simulink model "gm_parallel_phase_voltages_per_switching_state_6"  (R2022a)
settings: Solver=FixedStepDiscrete  StartTime=0.0  StopTime=10.0  RelTol=1e-3
undefined symbols (not defined in the file or in its folder): f_c, u_dc
libraries: hdlmdlgenlib x82
(part 4 of 5)

== system gm_parallel_phase_voltages_per_switching_state_6/Phase_voltages_per_switching_state/Subsystem/MATLAB Function7 ==
  theta_el_with_offset : Inport  OutDataTypeStr=single  PortDimensions=1  SampleTime=1e-08
  u_dc_link_voltage : Inport  Port=2  OutDataTypeStr=single  PortDimensions=1  SampleTime=1e-08
  Index : Inport  Port=3  OutDataTypeStr=int32  PortDimensions=1  SampleTime=1e-08
  Assignment : Assignment  NumberOfDimensions=2  SampleTime=1e-08  IndexOptions=Index vector (dialog),Index vector (dialog)  Indices=double(2),double(1)  OutputSizes=double(0),double(0)
  Assignment1 : Assignment  NumberOfDimensions=2  SampleTime=1e-08  IndexOptions=Index vector (dialog),Index vector (dialog)  Indices=double(1),double(1)  OutputSizes=double(0),double(0)
  Assignment2 : Assignment  NumberOfDimensions=2  SampleTime=1e-08  IndexOptions=Index vector (dialog),Index vector (dialog)  Indices=double(4),double(1)  OutputSizes=double(0),double(0)
  Assignment3 : Assignment  NumberOfDimensions=2  SampleTime=1e-08  IndexOptions=Index vector (dialog),Index vector (dialog)  Indices=double(3),double(1)  OutputSizes=double(0),double(0)
  Selector : Selector  NumberOfDimensions=2  SampleTime=1e-08  IndexOptions=Index vector (dialog),Index vector (dialog)  Indices=double(1),double(1)  OutputSizes=double(0),double(0)
  Selector1 : Selector  NumberOfDimensions=2  SampleTime=1e-08  IndexOptions=Index vector (dialog),Index vector (dialog)  Indices=double(2),double(1)  OutputSizes=double(0),double(0)
  Selector2 : Selector  NumberOfDimensions=2  SampleTime=1e-08  IndexOptions=Index vector (dialog),Index vector (dialog)  Indices=double(3),double(1)  OutputSizes=double(0),double(0)
  Selector3 : Selector  NumberOfDimensions=2  SampleTime=1e-08  IndexOptions=Index vector (dialog),Index vector (dialog)  Indices=double(4),double(1)  OutputSizes=double(0),double(0)
  Selector4 : Selector  NumberOfDimensions=2  SampleTime=1e-08  IndexOptions=Index vector (dialog),Index vector (port)  Indices=double(2),double(-1)  OutputSizes=double(0),double(0)
  Selector5 : Selector  NumberOfDimensions=2  SampleTime=1e-08  IndexOptions=Index vector (dialog),Index vector (port)  Indices=double(1),double(-1)  OutputSizes=double(0),double(0)
  Selector6 : Selector  NumberOfDimensions=2  SampleTime=1e-08  IndexOptions=Index vector (dialog),Index vector (port)  Indices=double(4),double(-1)  OutputSizes=double(0),double(0)
  Selector7 : Selector  NumberOfDimensions=2  SampleTime=1e-08  IndexOptions=Index vector (dialog),Index vector (port)  Indices=double(2),double(-1)  OutputSizes=double(0),double(0)
  Selector8 : Selector  NumberOfDimensions=2  SampleTime=1e-08  IndexOptions=Index vector (dialog),Index vector (port)  Indices=double(1),double(-1)  OutputSizes=double(0),double(0)
  Selector9 : Selector  NumberOfDimensions=2  SampleTime=1e-08  IndexOptions=Index vector (dialog),Index vector (port)  Indices=double(3),double(-1)  OutputSizes=double(0),double(0)
  adder : Sum  AccumDataTypeStr=int32  OutDataTypeStr=int32  RndMeth=Nearest  SaturateOnIntegerOverflow=on  SampleTime=1e-08
  adder1 : Subsystem
      mask Display: disp('NFP\nadd');
  adder2 : Subsystem
      mask Display: disp('NFP\nadd');
  const{,1..2,5..7} (6 alike) : Constant  Value=single([0 -0.3333333432674408 0 -0.3333333432674408 0.3333333432674408 -0.3333333432674408 0.3333333432674408 -0.3333333432674408 -0.1666666716337204 -0.044658198952674866 -0.1666666716337204 -0.6220084428787231 0.1666666716337204 -0.044658198952674866 0.1666666716337204 -0.6220084428787231]).'  VectorParams1D=off  OutDataTypeStr=single  SampleTime=1e-08
  const3 : Constant  Value="repmat(single(0),[4  1])"  VectorParams1D=off  OutDataTypeStr=single  SampleTime=1e-08
  const4 : Constant  VectorParams1D=off  OutDataTypeStr=int32  SampleTime=1e-08
  cos_to_sincos : Subsystem
      mask Display: disp('NFP\ntrig2');
  cos_to_sincos_out1_buff : hdlmdlgenlib/Buffer
      settings: SourceProductBaseCode=SL
  cos_to_sincos_out2_buff : hdlmdlgenlib/Buffer
      settings: SourceProductBaseCode=SL
  delayMatch{,1,3..4} (4 alike) : Delay  DelayLength=double(27)  InitialCondition=0  SampleTime=1e-08
  delayMatch{6..11} (6 alike) : Delay  DelayLength=double(2)  InitialCondition=0  SampleTime=1e-08
  delayMatch{12..17} (6 alike) : Delay  DelayLength=double(16)  InitialCondition=0  SampleTime=1e-08
  delayMatch2 : Delay  DelayLength=double(39)  InitialCondition=0  SampleTime=1e-08
  delayMatch5 : Delay  DelayLength=double(39)  InitialCondition=0  SampleTime=1e-08
  multiplier : Subsystem
      mask Display: disp('NFP\nmul');
  multiplier1 : Subsystem
      mask Display: disp('NFP\nmul');
  multiplier2 : Subsystem
      mask Display: disp('NFP\nmul');
  multiplier3 : Subsystem
      mask Display: disp('NFP\nmul');
  multiplier4 : Subsystem
      mask Display: disp('NFP\nmul');
  multiplier_outbuff : hdlmdlgenlib/Buffer
      settings: SourceProductBaseCode=SL
  t{,1..5} (6 alike) : Reshape  OutputDimensionality=Customize  OutputDimensions=[4,4]
  t6 : Mux
  uminus : Subsystem
      mask Display: disp('NFP\numinus');
  d_voltage_per_switching_state : Outport  SampleTime=1e-08  VectorParamsAs1DForOutWhenUnconnected=off
  q_voltage_per_switching_state : Outport  Port=2  SampleTime=1e-08
  x_voltage_per_switching_state : Outport  Port=3  SampleTime=1e-08
  y_voltage_per_switching_state : Outport  Port=4  SampleTime=1e-08
  wires:
  Selector/1 -> d_voltage_per_switching_state/1
  Selector1/1 -> q_voltage_per_switching_state/1
  Selector2/1 -> x_voltage_per_switching_state/1
  Selector3/1 -> y_voltage_per_switching_state/1
  multiplier_outbuff/1 -> Selector3/1, Selector2/1, Selector1/1, Selector/1
  Assignment/1 -> multiplier/2(In2)
  Assignment1/1 -> Assignment/1
  delayMatch14/1 -> Assignment1/1
  delayMatch16/1 -> multiplier1/2(In2)
  cos_to_sincos_out2_buff/1 -> multiplier4/1(In1), multiplier1/1(In1)
  delayMatch15/1 -> multiplier2/2(In2)
  Selector6/1 -> Assignment2/2
  Assignment3/1 -> Assignment2/1
  adder/1 -> Selector9/2, Selector8/2, Selector7/2, Selector6/2, Selector5/2, Selector4/2
  t/1 -> Selector4/1
  t1/1 -> Selector5/1
  cos_to_sincos_out1_buff/1 -> multiplier3/1(In1), uminus/1(In1)
  delayMatch13/1 -> multiplier3/2(In2)
  delayMatch12/1 -> multiplier4/2(In2)
  t2/1 -> Selector6/1
  Selector9/1 -> Assignment3/2
  const3/1 -> Assignment3/1
  const4/1 -> adder/2
  t3/1 -> Selector7/1
  t4/1 -> Selector8/1
  t5/1 -> Selector9/1
  const/1 -> t/1
  const1/1 -> t1/1
  const2/1 -> t2/1
  const5/1 -> t3/1
  const6/1 -> t4/1
  const7/1 -> t5/1
  delayMatch17/1 -> multiplier/1(In1)
  multiplier/1(Out1) -> multiplier_outbuff/1
  adder1/1(Out1) -> Assignment/2
  multiplier1/1(Out1) -> adder1/2(In2)
  multiplier2/1(Out1) -> adder1/1(In1)
  adder2/1(Out1) -> Assignment1/2
  uminus/1(Out1) -> multiplier2/1(In1)
  multiplier3/1(Out1) -> adder2/2(In2)
  multiplier4/1(Out1) -> adder2/1(In1)
  cos_to_sincos/1(Out1) -> cos_to_sincos_out1_buff/1
  cos_to_sincos/2(Out2) -> cos_to_sincos_out2_buff/1
  Selector8/1 -> delayMatch/1
  Selector7/1 -> delayMatch1/1
  Assignment2/1 -> delayMatch2/1
  Selector5/1 -> delayMatch3/1
  Selector4/1 -> delayMatch4/1
  t6/1 -> delayMatch5/1
  delayMatch/1 -> delayMatch6/1
  delayMatch1/1 -> delayMatch7/1
  delayMatch2/1 -> delayMatch8/1
  delayMatch3/1 -> delayMatch9/1
  delayMatch4/1 -> delayMatch10/1
  delayMatch5/1 -> delayMatch11/1
  delayMatch6/1 -> delayMatch12/1
  delayMatch7/1 -> delayMatch13/1
  delayMatch8/1 -> delayMatch14/1
  delayMatch9/1 -> delayMatch15/1
  delayMatch10/1 -> delayMatch16/1
  delayMatch11/1 -> delayMatch17/1
  theta_el_with_offset/1 -> cos_to_sincos/1(In1)
  u_dc_link_voltage/1 -> t6/4, t6/3, t6/2, t6/1
  Index/1 -> adder/1

== system gm_parallel_phase_voltages_per_switching_state_6/Phase_voltages_per_switching_state/Subsystem/MATLAB Function8 ==
  theta_el_with_offset : Inport  OutDataTypeStr=single  PortDimensions=1  SampleTime=1e-08
  u_dc_link_voltage : Inport  Port=2  OutDataTypeStr=single  PortDimensions=1  SampleTime=1e-08
  Index : Inport  Port=3  OutDataTypeStr=int32  PortDimensions=1  SampleTime=1e-08
  Assignment : Assignment  NumberOfDimensions=2  SampleTime=1e-08  IndexOptions=Index vector (dialog),Index vector (dialog)  Indices=double(2),double(1)  OutputSizes=double(0),double(0)
  Assignment1 : Assignment  NumberOfDimensions=2  SampleTime=1e-08  IndexOptions=Index vector (dialog),Index vector (dialog)  Indices=double(1),double(1)  OutputSizes=double(0),double(0)
  Assignment2 : Assignment  NumberOfDimensions=2  SampleTime=1e-08  IndexOptions=Index vector (dialog),Index vector (dialog)  Indices=double(4),double(1)  OutputSizes=double(0),double(0)
  Assignment3 : Assignment  NumberOfDimensions=2  SampleTime=1e-08  IndexOptions=Index vector (dialog),Index vector (dialog)  Indices=double(3),double(1)  OutputSizes=double(0),double(0)
  Selector : Selector  NumberOfDimensions=2  SampleTime=1e-08  IndexOptions=Index vector (dialog),Index vector (dialog)  Indices=double(1),double(1)  OutputSizes=double(0),double(0)
  Selector1 : Selector  NumberOfDimensions=2  SampleTime=1e-08  IndexOptions=Index vector (dialog),Index vector (dialog)  Indices=double(2),double(1)  OutputSizes=double(0),double(0)
  Selector2 : Selector  NumberOfDimensions=2  SampleTime=1e-08  IndexOptions=Index vector (dialog),Index vector (dialog)  Indices=double(3),double(1)  OutputSizes=double(0),double(0)
  Selector3 : Selector  NumberOfDimensions=2  SampleTime=1e-08  IndexOptions=Index vector (dialog),Index vector (dialog)  Indices=double(4),double(1)  OutputSizes=double(0),double(0)
  Selector4 : Selector  NumberOfDimensions=2  SampleTime=1e-08  IndexOptions=Index vector (dialog),Index vector (port)  Indices=double(2),double(-1)  OutputSizes=double(0),double(0)
  Selector5 : Selector  NumberOfDimensions=2  SampleTime=1e-08  IndexOptions=Index vector (dialog),Index vector (port)  Indices=double(1),double(-1)  OutputSizes=double(0),double(0)
  Selector6 : Selector  NumberOfDimensions=2  SampleTime=1e-08  IndexOptions=Index vector (dialog),Index vector (port)  Indices=double(4),double(-1)  OutputSizes=double(0),double(0)
  Selector7 : Selector  NumberOfDimensions=2  SampleTime=1e-08  IndexOptions=Index vector (dialog),Index vector (port)  Indices=double(2),double(-1)  OutputSizes=double(0),double(0)
  Selector8 : Selector  NumberOfDimensions=2  SampleTime=1e-08  IndexOptions=Index vector (dialog),Index vector (port)  Indices=double(1),double(-1)  OutputSizes=double(0),double(0)
  Selector9 : Selector  NumberOfDimensions=2  SampleTime=1e-08  IndexOptions=Index vector (dialog),Index vector (port)  Indices=double(3),double(-1)  OutputSizes=double(0),double(0)
  adder : Sum  AccumDataTypeStr=int32  OutDataTypeStr=int32  RndMeth=Nearest  SaturateOnIntegerOverflow=on  SampleTime=1e-08
  adder1 : Subsystem
      mask Display: disp('NFP\nadd');
  adder2 : Subsystem
      mask Display: disp('NFP\nadd');
  const{,1..2,5..7} (6 alike) : Constant  Value=single([-0.1666666716337204 0.044658198952674866 -0.1666666716337204 0.6220084428787231 0.1666666716337204 0.044658198952674866 0.1666666716337204 0.6220084428787231 -0.3333333432674408 0.3333333432674408 -0.3333333432674408 0.3333333432674408 0 0.3333333432674408 0 0.3333333432674408]).'  VectorParams1D=off  OutDataTypeStr=single  SampleTime=1e-08
  const3 : Constant  Value="repmat(single(0),[4  1])"  VectorParams1D=off  OutDataTypeStr=single  SampleTime=1e-08
  const4 : Constant  VectorParams1D=off  OutDataTypeStr=int32  SampleTime=1e-08
  cos_to_sincos : Subsystem
      mask Display: disp('NFP\ntrig2');
  cos_to_sincos_out1_buff : hdlmdlgenlib/Buffer
      settings: SourceProductBaseCode=SL
  cos_to_sincos_out2_buff : hdlmdlgenlib/Buffer
      settings: SourceProductBaseCode=SL
  delayMatch{,1,3..4} (4 alike) : Delay  DelayLength=double(27)  InitialCondition=0  SampleTime=1e-08
  delayMatch{6..11} (6 alike) : Delay  DelayLength=double(2)  InitialCondition=0  SampleTime=1e-08
  delayMatch{12..17} (6 alike) : Delay  DelayLength=double(16)  InitialCondition=0  SampleTime=1e-08
  delayMatch2 : Delay  DelayLength=double(39)  InitialCondition=0  SampleTime=1e-08
  delayMatch5 : Delay  DelayLength=double(39)  InitialCondition=0  SampleTime=1e-08
  multiplier : Subsystem
      mask Display: disp('NFP\nmul');
  multiplier1 : Subsystem
      mask Display: disp('NFP\nmul');
  multiplier2 : Subsystem
      mask Display: disp('NFP\nmul');
  multiplier3 : Subsystem
      mask Display: disp('NFP\nmul');
  multiplier4 : Subsystem
      mask Display: disp('NFP\nmul');
  multiplier_outbuff : hdlmdlgenlib/Buffer
      settings: SourceProductBaseCode=SL
  t{,1..5} (6 alike) : Reshape  OutputDimensionality=Customize  OutputDimensions=[4,4]
  t6 : Mux
  uminus : Subsystem
      mask Display: disp('NFP\numinus');
  d_voltage_per_switching_state : Outport  SampleTime=1e-08  VectorParamsAs1DForOutWhenUnconnected=off
  q_voltage_per_switching_state : Outport  Port=2  SampleTime=1e-08
  x_voltage_per_switching_state : Outport  Port=3  SampleTime=1e-08
  y_voltage_per_switching_state : Outport  Port=4  SampleTime=1e-08
  wires:
  Selector/1 -> d_voltage_per_switching_state/1
  Selector1/1 -> q_voltage_per_switching_state/1
  Selector2/1 -> x_voltage_per_switching_state/1
  Selector3/1 -> y_voltage_per_switching_state/1
  multiplier_outbuff/1 -> Selector3/1, Selector2/1, Selector1/1, Selector/1
  Assignment/1 -> multiplier/2(In2)
  Assignment1/1 -> Assignment/1
  delayMatch14/1 -> Assignment1/1
  delayMatch16/1 -> multiplier1/2(In2)
  cos_to_sincos_out2_buff/1 -> multiplier4/1(In1), multiplier1/1(In1)
  delayMatch15/1 -> multiplier2/2(In2)
  Selector6/1 -> Assignment2/2
  Assignment3/1 -> Assignment2/1
  adder/1 -> Selector9/2, Selector8/2, Selector7/2, Selector6/2, Selector5/2, Selector4/2
  t/1 -> Selector4/1
  t1/1 -> Selector5/1
  cos_to_sincos_out1_buff/1 -> multiplier3/1(In1), uminus/1(In1)
  delayMatch13/1 -> multiplier3/2(In2)
  delayMatch12/1 -> multiplier4/2(In2)
  t2/1 -> Selector6/1
  Selector9/1 -> Assignment3/2
  const3/1 -> Assignment3/1
  const4/1 -> adder/2
  t3/1 -> Selector7/1
  t4/1 -> Selector8/1
  t5/1 -> Selector9/1
  const/1 -> t/1
  const1/1 -> t1/1
  const2/1 -> t2/1
  const5/1 -> t3/1
  const6/1 -> t4/1
  const7/1 -> t5/1
  delayMatch17/1 -> multiplier/1(In1)
  multiplier/1(Out1) -> multiplier_outbuff/1
  adder1/1(Out1) -> Assignment/2
  multiplier1/1(Out1) -> adder1/2(In2)
  multiplier2/1(Out1) -> adder1/1(In1)
  adder2/1(Out1) -> Assignment1/2
  uminus/1(Out1) -> multiplier2/1(In1)
  multiplier3/1(Out1) -> adder2/2(In2)
  multiplier4/1(Out1) -> adder2/1(In1)
  cos_to_sincos/1(Out1) -> cos_to_sincos_out1_buff/1
  cos_to_sincos/2(Out2) -> cos_to_sincos_out2_buff/1
  Selector8/1 -> delayMatch/1
  Selector7/1 -> delayMatch1/1
  Assignment2/1 -> delayMatch2/1
  Selector5/1 -> delayMatch3/1
  Selector4/1 -> delayMatch4/1
  t6/1 -> delayMatch5/1
  delayMatch/1 -> delayMatch6/1
  delayMatch1/1 -> delayMatch7/1
  delayMatch2/1 -> delayMatch8/1
  delayMatch3/1 -> delayMatch9/1
  delayMatch4/1 -> delayMatch10/1
  delayMatch5/1 -> delayMatch11/1
  delayMatch6/1 -> delayMatch12/1
  delayMatch7/1 -> delayMatch13/1
  delayMatch8/1 -> delayMatch14/1
  delayMatch9/1 -> delayMatch15/1
  delayMatch10/1 -> delayMatch16/1
  delayMatch11/1 -> delayMatch17/1
  theta_el_with_offset/1 -> cos_to_sincos/1(In1)
  u_dc_link_voltage/1 -> t6/4, t6/3, t6/2, t6/1
  Index/1 -> adder/1

== system gm_parallel_phase_voltages_per_switching_state_6/Phase_voltages_per_switching_state/Subsystem/MATLAB Function9 ==
  theta_el_with_offset : Inport  OutDataTypeStr=single  PortDimensions=1  SampleTime=1e-08
  u_dc_link_voltage : Inport  Port=2  OutDataTypeStr=single  PortDimensions=1  SampleTime=1e-08
  Index : Inport  Port=3  OutDataTypeStr=int32  PortDimensions=1  SampleTime=1e-08
  Assignment : Assignment  NumberOfDimensions=2  SampleTime=1e-08  IndexOptions=Index vector (dialog),Index vector (dialog)  Indices=double(2),double(1)  OutputSizes=double(0),double(0)
  Assignment1 : Assignment  NumberOfDimensions=2  SampleTime=1e-08  IndexOptions=Index vector (dialog),Index vector (dialog)  Indices=double(1),double(1)  OutputSizes=double(0),double(0)
  Assignment2 : Assignment  NumberOfDimensions=2  SampleTime=1e-08  IndexOptions=Index vector (dialog),Index vector (dialog)  Indices=double(4),double(1)  OutputSizes=double(0),double(0)
  Assignment3 : Assignment  NumberOfDimensions=2  SampleTime=1e-08  IndexOptions=Index vector (dialog),Index vector (dialog)  Indices=double(3),double(1)  OutputSizes=double(0),double(0)
  Selector : Selector  NumberOfDimensions=2  SampleTime=1e-08  IndexOptions=Index vector (dialog),Index vector (dialog)  Indices=double(1),double(1)  OutputSizes=double(0),double(0)
  Selector1 : Selector  NumberOfDimensions=2  SampleTime=1e-08  IndexOptions=Index vector (dialog),Index vector (dialog)  Indices=double(2),double(1)  OutputSizes=double(0),double(0)
  Selector2 : Selector  NumberOfDimensions=2  SampleTime=1e-08  IndexOptions=Index vector (dialog),Index vector (dialog)  Indices=double(3),double(1)  OutputSizes=double(0),double(0)
  Selector3 : Selector  NumberOfDimensions=2  SampleTime=1e-08  IndexOptions=Index vector (dialog),Index vector (dialog)  Indices=double(4),double(1)  OutputSizes=double(0),double(0)
  Selector4 : Selector  NumberOfDimensions=2  SampleTime=1e-08  IndexOptions=Index vector (dialog),Index vector (port)  Indices=double(2),double(-1)  OutputSizes=double(0),double(0)
  Selector5 : Selector  NumberOfDimensions=2  SampleTime=1e-08  IndexOptions=Index vector (dialog),Index vector (port)  Indices=double(1),double(-1)  OutputSizes=double(0),double(0)
  Selector6 : Selector  NumberOfDimensions=2  SampleTime=1e-08  IndexOptions=Index vector (dialog),Index vector (port)  Indices=double(4),double(-1)  OutputSizes=double(0),double(0)
  Selector7 : Selector  NumberOfDimensions=2  SampleTime=1e-08  IndexOptions=Index vector (dialog),Index vector (port)  Indices=double(2),double(-1)  OutputSizes=double(0),double(0)
  Selector8 : Selector  NumberOfDimensions=2  SampleTime=1e-08  IndexOptions=Index vector (dialog),Index vector (port)  Indices=double(1),double(-1)  OutputSizes=double(0),double(0)
  Selector9 : Selector  NumberOfDimensions=2  SampleTime=1e-08  IndexOptions=Index vector (dialog),Index vector (port)  Indices=double(3),double(-1)  OutputSizes=double(0),double(0)
  adder : Sum  AccumDataTypeStr=int32  OutDataTypeStr=int32  RndMeth=Nearest  SaturateOnIntegerOverflow=on  SampleTime=1e-08
  adder1 : Subsystem
      mask Display: disp('NFP\nadd');
  adder2 : Subsystem
      mask Display: disp('NFP\nadd');
  const{,1..2,5..7} (6 alike) : Constant  Value=single([0 0.3333333432674408 0 0.3333333432674408 0.3333333432674408 0.3333333432674408 0.3333333432674408 0.3333333432674408 -0.1666666716337204 0.6220084428787231 -0.1666666716337204 0.044658198952674866 0.1666666716337204 0.6220084428787231 0.1666666716337204 0.044658198952674866]).'  VectorParams1D=off  OutDataTypeStr=single  SampleTime=1e-08
  const3 : Constant  Value="repmat(single(0),[4  1])"  VectorParams1D=off  OutDataTypeStr=single  SampleTime=1e-08
  const4 : Constant  VectorParams1D=off  OutDataTypeStr=int32  SampleTime=1e-08
  cos_to_sincos : Subsystem
      mask Display: disp('NFP\ntrig2');
  cos_to_sincos_out1_buff : hdlmdlgenlib/Buffer
      settings: SourceProductBaseCode=SL
  cos_to_sincos_out2_buff : hdlmdlgenlib/Buffer
      settings: SourceProductBaseCode=SL
  delayMatch{,1,3..4} (4 alike) : Delay  DelayLength=double(27)  InitialCondition=0  SampleTime=1e-08
  delayMatch{6..11} (6 alike) : Delay  DelayLength=double(2)  InitialCondition=0  SampleTime=1e-08
  delayMatch{12..17} (6 alike) : Delay  DelayLength=double(16)  InitialCondition=0  SampleTime=1e-08
  delayMatch2 : Delay  DelayLength=double(39)  InitialCondition=0  SampleTime=1e-08
  delayMatch5 : Delay  DelayLength=double(39)  InitialCondition=0  SampleTime=1e-08
  multiplier : Subsystem
      mask Display: disp('NFP\nmul');
  multiplier1 : Subsystem
      mask Display: disp('NFP\nmul');
  multiplier2 : Subsystem
      mask Display: disp('NFP\nmul');
  multiplier3 : Subsystem
      mask Display: disp('NFP\nmul');
  multiplier4 : Subsystem
      mask Display: disp('NFP\nmul');
  multiplier_outbuff : hdlmdlgenlib/Buffer
      settings: SourceProductBaseCode=SL
  t{,1..5} (6 alike) : Reshape  OutputDimensionality=Customize  OutputDimensions=[4,4]
  t6 : Mux
  uminus : Subsystem
      mask Display: disp('NFP\numinus');
  d_voltage_per_switching_state : Outport  SampleTime=1e-08  VectorParamsAs1DForOutWhenUnconnected=off
  q_voltage_per_switching_state : Outport  Port=2  SampleTime=1e-08
  x_voltage_per_switching_state : Outport  Port=3  SampleTime=1e-08
  y_voltage_per_switching_state : Outport  Port=4  SampleTime=1e-08
  wires:
  Selector/1 -> d_voltage_per_switching_state/1
  Selector1/1 -> q_voltage_per_switching_state/1
  Selector2/1 -> x_voltage_per_switching_state/1
  Selector3/1 -> y_voltage_per_switching_state/1
  multiplier_outbuff/1 -> Selector3/1, Selector2/1, Selector1/1, Selector/1
  Assignment/1 -> multiplier/2(In2)
  Assignment1/1 -> Assignment/1
  delayMatch14/1 -> Assignment1/1
  delayMatch16/1 -> multiplier1/2(In2)
  cos_to_sincos_out2_buff/1 -> multiplier4/1(In1), multiplier1/1(In1)
  delayMatch15/1 -> multiplier2/2(In2)
  Selector6/1 -> Assignment2/2
  Assignment3/1 -> Assignment2/1
  adder/1 -> Selector9/2, Selector8/2, Selector7/2, Selector6/2, Selector5/2, Selector4/2
  t/1 -> Selector4/1
  t1/1 -> Selector5/1
  cos_to_sincos_out1_buff/1 -> multiplier3/1(In1), uminus/1(In1)
  delayMatch13/1 -> multiplier3/2(In2)
  delayMatch12/1 -> multiplier4/2(In2)
  t2/1 -> Selector6/1
  Selector9/1 -> Assignment3/2
  const3/1 -> Assignment3/1
  const4/1 -> adder/2
  t3/1 -> Selector7/1
  t4/1 -> Selector8/1
  t5/1 -> Selector9/1
  const/1 -> t/1
  const1/1 -> t1/1
  const2/1 -> t2/1
  const5/1 -> t3/1
  const6/1 -> t4/1
  const7/1 -> t5/1
  delayMatch17/1 -> multiplier/1(In1)
  multiplier/1(Out1) -> multiplier_outbuff/1
  adder1/1(Out1) -> Assignment/2
  multiplier1/1(Out1) -> adder1/2(In2)
  multiplier2/1(Out1) -> adder1/1(In1)
  adder2/1(Out1) -> Assignment1/2
  uminus/1(Out1) -> multiplier2/1(In1)
  multiplier3/1(Out1) -> adder2/2(In2)
  multiplier4/1(Out1) -> adder2/1(In1)
  cos_to_sincos/1(Out1) -> cos_to_sincos_out1_buff/1
  cos_to_sincos/2(Out2) -> cos_to_sincos_out2_buff/1
  Selector8/1 -> delayMatch/1
  Selector7/1 -> delayMatch1/1
  Assignment2/1 -> delayMatch2/1
  Selector5/1 -> delayMatch3/1
  Selector4/1 -> delayMatch4/1
  t6/1 -> delayMatch5/1
  delayMatch/1 -> delayMatch6/1
  delayMatch1/1 -> delayMatch7/1
  delayMatch2/1 -> delayMatch8/1
  delayMatch3/1 -> delayMatch9/1
  delayMatch4/1 -> delayMatch10/1
  delayMatch5/1 -> delayMatch11/1
  delayMatch6/1 -> delayMatch12/1
  delayMatch7/1 -> delayMatch13/1
  delayMatch8/1 -> delayMatch14/1
  delayMatch9/1 -> delayMatch15/1
  delayMatch10/1 -> delayMatch16/1
  delayMatch11/1 -> delayMatch17/1
  theta_el_with_offset/1 -> cos_to_sincos/1(In1)
  u_dc_link_voltage/1 -> t6/4, t6/3, t6/2, t6/1
  Index/1 -> adder/1

== system gm_parallel_phase_voltages_per_switching_state_6/Phase_voltages_per_switching_state/Subsystem/MATLAB Function/adder1 ==
  In1 : Inport
  In2 : Inport  Port=2
  adder1 : Sum  OutDataTypeStr=single  SampleTime=1e-08
  adder1_pd1 : Delay  DelayLength=6
  Out1 : Outport
  wires:
  In1/1 -> adder1/1
  In2/1 -> adder1/2
  adder1/1 -> adder1_pd1/1
  adder1_pd1/1 -> Out1/1

== system gm_parallel_phase_voltages_per_switching_state_6/Phase_voltages_per_switching_state/Subsystem/MATLAB Function/adder2 ==
  In1 : Inport
  In2 : Inport  Port=2
  adder2 : Sum  OutDataTypeStr=single  SampleTime=1e-08
  adder2_pd1 : Delay  DelayLength=6
  Out1 : Outport
  wires:
  In1/1 -> adder2/1
  In2/1 -> adder2/2
  adder2/1 -> adder2_pd1/1
  adder2_pd1/1 -> Out1/1

== system gm_parallel_phase_voltages_per_switching_state_6/Phase_voltages_per_switching_state/Subsystem/MATLAB Function/cos_to_sincos ==
  In1 : Inport
  cos_to_sincos : Trigonometry  Operator=sincos  SampleTime=1e-08
  cos_to_sincos_pd1 : Delay  DelayLength=27
  cos_to_sincos_pd2 : Delay  DelayLength=27
  Out1 : Outport
  Out2 : Outport  Port=2
  wires:
  In1/1 -> cos_to_sincos/1
  cos_to_sincos/1 -> cos_to_sincos_pd1/1
  cos_to_sincos_pd1/1 -> Out1/1
  cos_to_sincos/2 -> cos_to_sincos_pd2/1
  cos_to_sincos_pd2/1 -> Out2/1

== system gm_parallel_phase_voltages_per_switching_state_6/Phase_voltages_per_switching_state/Subsystem/MATLAB Function/multiplier ==
  In1 : Inport
  In2 : Inport  Port=2
  multiplier : Product  Inputs=**  OutDataTypeStr=single  SampleTime=1e-08
  multiplier_pd1 : Delay  DelayLength=6
  Out1 : Outport
  wires:
  In1/1 -> multiplier/1
  In2/1 -> multiplier/2
  multiplier/1 -> multiplier_pd1/1
  multiplier_pd1/1 -> Out1/1

== system gm_parallel_phase_voltages_per_switching_state_6/Phase_voltages_per_switching_state/Subsystem/MATLAB Function/multiplier1 ==
  In1 : Inport
  In2 : Inport  Port=2
  multiplier1 : Product  Inputs=**  OutDataTypeStr=single  SampleTime=1e-08
  multiplier1_pd1 : Delay  DelayLength=6
  Out1 : Outport
  wires:
  In1/1 -> multiplier1/1
  In2/1 -> multiplier1/2
  multiplier1/1 -> multiplier1_pd1/1
  multiplier1_pd1/1 -> Out1/1

== system gm_parallel_phase_voltages_per_switching_state_6/Phase_voltages_per_switching_state/Subsystem/MATLAB Function/multiplier2 ==
  In1 : Inport
  In2 : Inport  Port=2
  multiplier2 : Product  Inputs=**  OutDataTypeStr=single  SampleTime=1e-08
  multiplier2_pd1 : Delay  DelayLength=6
  Out1 : Outport
  wires:
  In1/1 -> multiplier2/1
  In2/1 -> multiplier2/2
  multiplier2/1 -> multiplier2_pd1/1
  multiplier2_pd1/1 -> Out1/1

== system gm_parallel_phase_voltages_per_switching_state_6/Phase_voltages_per_switching_state/Subsystem/MATLAB Function/multiplier3 ==
  In1 : Inport
  In2 : Inport  Port=2
  multiplier3 : Product  Inputs=**  OutDataTypeStr=single  SampleTime=1e-08
  multiplier3_pd1 : Delay  DelayLength=6
  Out1 : Outport
  wires:
  In1/1 -> multiplier3/1
  In2/1 -> multiplier3/2
  multiplier3/1 -> multiplier3_pd1/1
  multiplier3_pd1/1 -> Out1/1

== system gm_parallel_phase_voltages_per_switching_state_6/Phase_voltages_per_switching_state/Subsystem/MATLAB Function/multiplier4 ==
  In1 : Inport
  In2 : Inport  Port=2
  multiplier4 : Product  Inputs=**  OutDataTypeStr=single  SampleTime=1e-08
  multiplier4_pd1 : Delay  DelayLength=6
  Out1 : Outport
  wires:
  In1/1 -> multiplier4/1
  In2/1 -> multiplier4/2
  multiplier4/1 -> multiplier4_pd1/1
  multiplier4_pd1/1 -> Out1/1

== system gm_parallel_phase_voltages_per_switching_state_6/Phase_voltages_per_switching_state/Subsystem/MATLAB Function/uminus ==
  In1 : Inport
  uminus : UnaryMinus  SampleTime=1e-08
  Out1 : Outport
  wires:
  In1/1 -> uminus/1
  uminus/1 -> Out1/1

== system gm_parallel_phase_voltages_per_switching_state_6/Phase_voltages_per_switching_state/Subsystem/MATLAB Function1/adder1 ==
  In1 : Inport
  In2 : Inport  Port=2
  adder1 : Sum  OutDataTypeStr=single  SampleTime=1e-08
  adder1_pd1 : Delay  DelayLength=6
  Out1 : Outport
  wires:
  In1/1 -> adder1/1
  In2/1 -> adder1/2
  adder1/1 -> adder1_pd1/1
  adder1_pd1/1 -> Out1/1

== system gm_parallel_phase_voltages_per_switching_state_6/Phase_voltages_per_switching_state/Subsystem/MATLAB Function1/adder2 ==
  In1 : Inport
  In2 : Inport  Port=2
  adder2 : Sum  OutDataTypeStr=single  SampleTime=1e-08
  adder2_pd1 : Delay  DelayLength=6
  Out1 : Outport
  wires:
  In1/1 -> adder2/1
  In2/1 -> adder2/2
  adder2/1 -> adder2_pd1/1
  adder2_pd1/1 -> Out1/1

== system gm_parallel_phase_voltages_per_switching_state_6/Phase_voltages_per_switching_state/Subsystem/MATLAB Function1/cos_to_sincos ==
  In1 : Inport
  cos_to_sincos : Trigonometry  Operator=sincos  SampleTime=1e-08
  cos_to_sincos_pd1 : Delay  DelayLength=27
  cos_to_sincos_pd2 : Delay  DelayLength=27
  Out1 : Outport
  Out2 : Outport  Port=2
  wires:
  In1/1 -> cos_to_sincos/1
  cos_to_sincos/1 -> cos_to_sincos_pd1/1
  cos_to_sincos_pd1/1 -> Out1/1
  cos_to_sincos/2 -> cos_to_sincos_pd2/1
  cos_to_sincos_pd2/1 -> Out2/1

== system gm_parallel_phase_voltages_per_switching_state_6/Phase_voltages_per_switching_state/Subsystem/MATLAB Function1/multiplier ==
  In1 : Inport
  In2 : Inport  Port=2
  multiplier : Product  Inputs=**  OutDataTypeStr=single  SampleTime=1e-08
  multiplier_pd1 : Delay  DelayLength=6
  Out1 : Outport
  wires:
  In1/1 -> multiplier/1
  In2/1 -> multiplier/2
  multiplier/1 -> multiplier_pd1/1
  multiplier_pd1/1 -> Out1/1

== system gm_parallel_phase_voltages_per_switching_state_6/Phase_voltages_per_switching_state/Subsystem/MATLAB Function1/multiplier1 ==
  In1 : Inport
  In2 : Inport  Port=2
  multiplier1 : Product  Inputs=**  OutDataTypeStr=single  SampleTime=1e-08
  multiplier1_pd1 : Delay  DelayLength=6
  Out1 : Outport
  wires:
  In1/1 -> multiplier1/1
  In2/1 -> multiplier1/2
  multiplier1/1 -> multiplier1_pd1/1
  multiplier1_pd1/1 -> Out1/1

== system gm_parallel_phase_voltages_per_switching_state_6/Phase_voltages_per_switching_state/Subsystem/MATLAB Function1/multiplier2 ==
  In1 : Inport
  In2 : Inport  Port=2
  multiplier2 : Product  Inputs=**  OutDataTypeStr=single  SampleTime=1e-08
  multiplier2_pd1 : Delay  DelayLength=6
  Out1 : Outport
  wires:
  In1/1 -> multiplier2/1
  In2/1 -> multiplier2/2
  multiplier2/1 -> multiplier2_pd1/1
  multiplier2_pd1/1 -> Out1/1

== system gm_parallel_phase_voltages_per_switching_state_6/Phase_voltages_per_switching_state/Subsystem/MATLAB Function1/multiplier3 ==
  In1 : Inport
  In2 : Inport  Port=2
  multiplier3 : Product  Inputs=**  OutDataTypeStr=single  SampleTime=1e-08
  multiplier3_pd1 : Delay  DelayLength=6
  Out1 : Outport
  wires:
  In1/1 -> multiplier3/1
  In2/1 -> multiplier3/2
  multiplier3/1 -> multiplier3_pd1/1
  multiplier3_pd1/1 -> Out1/1

== system gm_parallel_phase_voltages_per_switching_state_6/Phase_voltages_per_switching_state/Subsystem/MATLAB Function1/multiplier4 ==
  In1 : Inport
  In2 : Inport  Port=2
  multiplier4 : Product  Inputs=**  OutDataTypeStr=single  SampleTime=1e-08
  multiplier4_pd1 : Delay  DelayLength=6
  Out1 : Outport
  wires:
  In1/1 -> multiplier4/1
  In2/1 -> multiplier4/2
  multiplier4/1 -> multiplier4_pd1/1
  multiplier4_pd1/1 -> Out1/1

== system gm_parallel_phase_voltages_per_switching_state_6/Phase_voltages_per_switching_state/Subsystem/MATLAB Function1/uminus ==
  In1 : Inport
  uminus : UnaryMinus  SampleTime=1e-08
  Out1 : Outport
  wires:
  In1/1 -> uminus/1
  uminus/1 -> Out1/1

== system gm_parallel_phase_voltages_per_switching_state_6/Phase_voltages_per_switching_state/Subsystem/MATLAB Function10/adder1 ==
  In1 : Inport
  In2 : Inport  Port=2
  adder1 : Sum  OutDataTypeStr=single  SampleTime=1e-08
  adder1_pd1 : Delay  DelayLength=6
  Out1 : Outport
  wires:
  In1/1 -> adder1/1
  In2/1 -> adder1/2
  adder1/1 -> adder1_pd1/1
  adder1_pd1/1 -> Out1/1

== system gm_parallel_phase_voltages_per_switching_state_6/Phase_voltages_per_switching_state/Subsystem/MATLAB Function10/adder2 ==
  In1 : Inport
  In2 : Inport  Port=2
  adder2 : Sum  OutDataTypeStr=single  SampleTime=1e-08
  adder2_pd1 : Delay  DelayLength=6
  Out1 : Outport
  wires:
  In1/1 -> adder2/1
  In2/1 -> adder2/2
  adder2/1 -> adder2_pd1/1
  adder2_pd1/1 -> Out1/1

== system gm_parallel_phase_voltages_per_switching_state_6/Phase_voltages_per_switching_state/Subsystem/MATLAB Function10/cos_to_sincos ==
  In1 : Inport
  cos_to_sincos : Trigonometry  Operator=sincos  SampleTime=1e-08
  cos_to_sincos_pd1 : Delay  DelayLength=27
  cos_to_sincos_pd2 : Delay  DelayLength=27
  Out1 : Outport
  Out2 : Outport  Port=2
  wires:
  In1/1 -> cos_to_sincos/1
  cos_to_sincos/1 -> cos_to_sincos_pd1/1
  cos_to_sincos_pd1/1 -> Out1/1
  cos_to_sincos/2 -> cos_to_sincos_pd2/1
  cos_to_sincos_pd2/1 -> Out2/1

== system gm_parallel_phase_voltages_per_switching_state_6/Phase_voltages_per_switching_state/Subsystem/MATLAB Function10/multiplier ==
  In1 : Inport
  In2 : Inport  Port=2
  multiplier : Product  Inputs=**  OutDataTypeStr=single  SampleTime=1e-08
  multiplier_pd1 : Delay  DelayLength=6
  Out1 : Outport
  wires:
  In1/1 -> multiplier/1
  In2/1 -> multiplier/2
  multiplier/1 -> multiplier_pd1/1
  multiplier_pd1/1 -> Out1/1

== system gm_parallel_phase_voltages_per_switching_state_6/Phase_voltages_per_switching_state/Subsystem/MATLAB Function10/multiplier1 ==
  In1 : Inport
  In2 : Inport  Port=2
  multiplier1 : Product  Inputs=**  OutDataTypeStr=single  SampleTime=1e-08
  multiplier1_pd1 : Delay  DelayLength=6
  Out1 : Outport
  wires:
  In1/1 -> multiplier1/1
  In2/1 -> multiplier1/2
  multiplier1/1 -> multiplier1_pd1/1
  multiplier1_pd1/1 -> Out1/1

== system gm_parallel_phase_voltages_per_switching_state_6/Phase_voltages_per_switching_state/Subsystem/MATLAB Function10/multiplier2 ==
  In1 : Inport
  In2 : Inport  Port=2
  multiplier2 : Product  Inputs=**  OutDataTypeStr=single  SampleTime=1e-08
  multiplier2_pd1 : Delay  DelayLength=6
  Out1 : Outport
  wires:
  In1/1 -> multiplier2/1
  In2/1 -> multiplier2/2
  multiplier2/1 -> multiplier2_pd1/1
  multiplier2_pd1/1 -> Out1/1

== system gm_parallel_phase_voltages_per_switching_state_6/Phase_voltages_per_switching_state/Subsystem/MATLAB Function10/multiplier3 ==
  In1 : Inport
  In2 : Inport  Port=2
  multiplier3 : Product  Inputs=**  OutDataTypeStr=single  SampleTime=1e-08
  multiplier3_pd1 : Delay  DelayLength=6
  Out1 : Outport
  wires:
  In1/1 -> multiplier3/1
  In2/1 -> multiplier3/2
  multiplier3/1 -> multiplier3_pd1/1
  multiplier3_pd1/1 -> Out1/1

== system gm_parallel_phase_voltages_per_switching_state_6/Phase_voltages_per_switching_state/Subsystem/MATLAB Function10/multiplier4 ==
  In1 : Inport
  In2 : Inport  Port=2
  multiplier4 : Product  Inputs=**  OutDataTypeStr=single  SampleTime=1e-08
  multiplier4_pd1 : Delay  DelayLength=6
  Out1 : Outport
  wires:
  In1/1 -> multiplier4/1
  In2/1 -> multiplier4/2
  multiplier4/1 -> multiplier4_pd1/1
  multiplier4_pd1/1 -> Out1/1

== system gm_parallel_phase_voltages_per_switching_state_6/Phase_voltages_per_switching_state/Subsystem/MATLAB Function10/uminus ==
  In1 : Inport
  uminus : UnaryMinus  SampleTime=1e-08
  Out1 : Outport
  wires:
  In1/1 -> uminus/1
  uminus/1 -> Out1/1

== system gm_parallel_phase_voltages_per_switching_state_6/Phase_voltages_per_switching_state/Subsystem/MATLAB Function11/adder1 ==
  In1 : Inport
  In2 : Inport  Port=2
  adder1 : Sum  OutDataTypeStr=single  SampleTime=1e-08
  adder1_pd1 : Delay  DelayLength=6
  Out1 : Outport
  wires:
  In1/1 -> adder1/1
  In2/1 -> adder1/2
  adder1/1 -> adder1_pd1/1
  adder1_pd1/1 -> Out1/1

== system gm_parallel_phase_voltages_per_switching_state_6/Phase_voltages_per_switching_state/Subsystem/MATLAB Function11/adder2 ==
  In1 : Inport
  In2 : Inport  Port=2
  adder2 : Sum  OutDataTypeStr=single  SampleTime=1e-08
  adder2_pd1 : Delay  DelayLength=6
  Out1 : Outport
  wires:
  In1/1 -> adder2/1
  In2/1 -> adder2/2
  adder2/1 -> adder2_pd1/1
  adder2_pd1/1 -> Out1/1

== system gm_parallel_phase_voltages_per_switching_state_6/Phase_voltages_per_switching_state/Subsystem/MATLAB Function11/cos_to_sincos ==
  In1 : Inport
  cos_to_sincos : Trigonometry  Operator=sincos  SampleTime=1e-08
  cos_to_sincos_pd1 : Delay  DelayLength=27
  cos_to_sincos_pd2 : Delay  DelayLength=27
  Out1 : Outport
  Out2 : Outport  Port=2
  wires:
  In1/1 -> cos_to_sincos/1
  cos_to_sincos/1 -> cos_to_sincos_pd1/1
  cos_to_sincos_pd1/1 -> Out1/1
  cos_to_sincos/2 -> cos_to_sincos_pd2/1
  cos_to_sincos_pd2/1 -> Out2/1

== system gm_parallel_phase_voltages_per_switching_state_6/Phase_voltages_per_switching_state/Subsystem/MATLAB Function11/multiplier ==
  In1 : Inport
  In2 : Inport  Port=2
  multiplier : Product  Inputs=**  OutDataTypeStr=single  SampleTime=1e-08
  multiplier_pd1 : Delay  DelayLength=6
  Out1 : Outport
  wires:
  In1/1 -> multiplier/1
  In2/1 -> multiplier/2
  multiplier/1 -> multiplier_pd1/1
  multiplier_pd1/1 -> Out1/1

== system gm_parallel_phase_voltages_per_switching_state_6/Phase_voltages_per_switching_state/Subsystem/MATLAB Function11/multiplier1 ==
  In1 : Inport
  In2 : Inport  Port=2
  multiplier1 : Product  Inputs=**  OutDataTypeStr=single  SampleTime=1e-08
  multiplier1_pd1 : Delay  DelayLength=6
  Out1 : Outport
  wires:
  In1/1 -> multiplier1/1
  In2/1 -> multiplier1/2
  multiplier1/1 -> multiplier1_pd1/1
  multiplier1_pd1/1 -> Out1/1

== system gm_parallel_phase_voltages_per_switching_state_6/Phase_voltages_per_switching_state/Subsystem/MATLAB Function11/multiplier2 ==
  In1 : Inport
  In2 : Inport  Port=2
  multiplier2 : Product  Inputs=**  OutDataTypeStr=single  SampleTime=1e-08
  multiplier2_pd1 : Delay  DelayLength=6
  Out1 : Outport
  wires:
  In1/1 -> multiplier2/1
  In2/1 -> multiplier2/2
  multiplier2/1 -> multiplier2_pd1/1
  multiplier2_pd1/1 -> Out1/1

== system gm_parallel_phase_voltages_per_switching_state_6/Phase_voltages_per_switching_state/Subsystem/MATLAB Function11/multiplier3 ==
  In1 : Inport
  In2 : Inport  Port=2
  multiplier3 : Product  Inputs=**  OutDataTypeStr=single  SampleTime=1e-08
  multiplier3_pd1 : Delay  DelayLength=6
  Out1 : Outport
  wires:
  In1/1 -> multiplier3/1
  In2/1 -> multiplier3/2
  multiplier3/1 -> multiplier3_pd1/1
  multiplier3_pd1/1 -> Out1/1

== system gm_parallel_phase_voltages_per_switching_state_6/Phase_voltages_per_switching_state/Subsystem/MATLAB Function11/multiplier4 ==
  In1 : Inport
  In2 : Inport  Port=2
  multiplier4 : Product  Inputs=**  OutDataTypeStr=single  SampleTime=1e-08
  multiplier4_pd1 : Delay  DelayLength=6
  Out1 : Outport
  wires:
  In1/1 -> multiplier4/1
  In2/1 -> multiplier4/2
  multiplier4/1 -> multiplier4_pd1/1
  multiplier4_pd1/1 -> Out1/1

== system gm_parallel_phase_voltages_per_switching_state_6/Phase_voltages_per_switching_state/Subsystem/MATLAB Function11/uminus ==
  In1 : Inport
  uminus : UnaryMinus  SampleTime=1e-08
  Out1 : Outport
  wires:
  In1/1 -> uminus/1
  uminus/1 -> Out1/1

== system gm_parallel_phase_voltages_per_switching_state_6/Phase_voltages_per_switching_state/Subsystem/MATLAB Function12/adder1 ==
  In1 : Inport
  In2 : Inport  Port=2
  adder1 : Sum  OutDataTypeStr=single  SampleTime=1e-08
  adder1_pd1 : Delay  DelayLength=6
  Out1 : Outport
  wires:
  In1/1 -> adder1/1
  In2/1 -> adder1/2
  adder1/1 -> adder1_pd1/1
  adder1_pd1/1 -> Out1/1

== system gm_parallel_phase_voltages_per_switching_state_6/Phase_voltages_per_switching_state/Subsystem/MATLAB Function12/adder2 ==
  In1 : Inport
  In2 : Inport  Port=2
  adder2 : Sum  OutDataTypeStr=single  SampleTime=1e-08
  adder2_pd1 : Delay  DelayLength=6
  Out1 : Outport
  wires:
  In1/1 -> adder2/1
  In2/1 -> adder2/2
  adder2/1 -> adder2_pd1/1
  adder2_pd1/1 -> Out1/1

== system gm_parallel_phase_voltages_per_switching_state_6/Phase_voltages_per_switching_state/Subsystem/MATLAB Function12/cos_to_sincos ==
  In1 : Inport
  cos_to_sincos : Trigonometry  Operator=sincos  SampleTime=1e-08
  cos_to_sincos_pd1 : Delay  DelayLength=27
  cos_to_sincos_pd2 : Delay  DelayLength=27
  Out1 : Outport
  Out2 : Outport  Port=2
  wires:
  In1/1 -> cos_to_sincos/1
  cos_to_sincos/1 -> cos_to_sincos_pd1/1
  cos_to_sincos_pd1/1 -> Out1/1
  cos_to_sincos/2 -> cos_to_sincos_pd2/1
  cos_to_sincos_pd2/1 -> Out2/1

== system gm_parallel_phase_voltages_per_switching_state_6/Phase_voltages_per_switching_state/Subsystem/MATLAB Function12/multiplier ==
  In1 : Inport
  In2 : Inport  Port=2
  multiplier : Product  Inputs=**  OutDataTypeStr=single  SampleTime=1e-08
  multiplier_pd1 : Delay  DelayLength=6
  Out1 : Outport
  wires:
  In1/1 -> multiplier/1
  In2/1 -> multiplier/2
  multiplier/1 -> multiplier_pd1/1
  multiplier_pd1/1 -> Out1/1

== system gm_parallel_phase_voltages_per_switching_state_6/Phase_voltages_per_switching_state/Subsystem/MATLAB Function12/multiplier1 ==
  In1 : Inport
  In2 : Inport  Port=2
  multiplier1 : Product  Inputs=**  OutDataTypeStr=single  SampleTime=1e-08
  multiplier1_pd1 : Delay  DelayLength=6
  Out1 : Outport
  wires:
  In1/1 -> multiplier1/1
  In2/1 -> multiplier1/2
  multiplier1/1 -> multiplier1_pd1/1
  multiplier1_pd1/1 -> Out1/1

== system gm_parallel_phase_voltages_per_switching_state_6/Phase_voltages_per_switching_state/Subsystem/MATLAB Function12/multiplier2 ==
  In1 : Inport
  In2 : Inport  Port=2
  multiplier2 : Product  Inputs=**  OutDataTypeStr=single  SampleTime=1e-08
  multiplier2_pd1 : Delay  DelayLength=6
  Out1 : Outport
  wires:
  In1/1 -> multiplier2/1
  In2/1 -> multiplier2/2
  multiplier2/1 -> multiplier2_pd1/1
  multiplier2_pd1/1 -> Out1/1

== system gm_parallel_phase_voltages_per_switching_state_6/Phase_voltages_per_switching_state/Subsystem/MATLAB Function12/multiplier3 ==
  In1 : Inport
  In2 : Inport  Port=2
  multiplier3 : Product  Inputs=**  OutDataTypeStr=single  SampleTime=1e-08
  multiplier3_pd1 : Delay  DelayLength=6
  Out1 : Outport
  wires:
  In1/1 -> multiplier3/1
  In2/1 -> multiplier3/2
  multiplier3/1 -> multiplier3_pd1/1
  multiplier3_pd1/1 -> Out1/1

== system gm_parallel_phase_voltages_per_switching_state_6/Phase_voltages_per_switching_state/Subsystem/MATLAB Function12/multiplier4 ==
  In1 : Inport
  In2 : Inport  Port=2
  multiplier4 : Product  Inputs=**  OutDataTypeStr=single  SampleTime=1e-08
  multiplier4_pd1 : Delay  DelayLength=6
  Out1 : Outport
  wires:
  In1/1 -> multiplier4/1
  In2/1 -> multiplier4/2
  multiplier4/1 -> multiplier4_pd1/1
  multiplier4_pd1/1 -> Out1/1

== system gm_parallel_phase_voltages_per_switching_state_6/Phase_voltages_per_switching_state/Subsystem/MATLAB Function12/uminus ==
  In1 : Inport
  uminus : UnaryMinus  SampleTime=1e-08
  Out1 : Outport
  wires:
  In1/1 -> uminus/1
  uminus/1 -> Out1/1

== system gm_parallel_phase_voltages_per_switching_state_6/Phase_voltages_per_switching_state/Subsystem/MATLAB Function13/adder1 ==
  In1 : Inport
  In2 : Inport  Port=2
  adder1 : Sum  OutDataTypeStr=single  SampleTime=1e-08
  adder1_pd1 : Delay  DelayLength=6
  Out1 : Outport
  wires:
  In1/1 -> adder1/1
  In2/1 -> adder1/2
  adder1/1 -> adder1_pd1/1
  adder1_pd1/1 -> Out1/1

== system gm_parallel_phase_voltages_per_switching_state_6/Phase_voltages_per_switching_state/Subsystem/MATLAB Function13/adder2 ==
  In1 : Inport
  In2 : Inport  Port=2
  adder2 : Sum  OutDataTypeStr=single  SampleTime=1e-08
  adder2_pd1 : Delay  DelayLength=6
  Out1 : Outport
  wires:
  In1/1 -> adder2/1
  In2/1 -> adder2/2
  adder2/1 -> adder2_pd1/1
  adder2_pd1/1 -> Out1/1

== system gm_parallel_phase_voltages_per_switching_state_6/Phase_voltages_per_switching_state/Subsystem/MATLAB Function13/cos_to_sincos ==
  In1 : Inport
  cos_to_sincos : Trigonometry  Operator=sincos  SampleTime=1e-08
  cos_to_sincos_pd1 : Delay  DelayLength=27
  cos_to_sincos_pd2 : Delay  DelayLength=27
  Out1 : Outport
  Out2 : Outport  Port=2
  wires:
  In1/1 -> cos_to_sincos/1
  cos_to_sincos/1 -> cos_to_sincos_pd1/1
  cos_to_sincos_pd1/1 -> Out1/1
  cos_to_sincos/2 -> cos_to_sincos_pd2/1
  cos_to_sincos_pd2/1 -> Out2/1

== system gm_parallel_phase_voltages_per_switching_state_6/Phase_voltages_per_switching_state/Subsystem/MATLAB Function13/multiplier ==
  In1 : Inport
  In2 : Inport  Port=2
  multiplier : Product  Inputs=**  OutDataTypeStr=single  SampleTime=1e-08
  multiplier_pd1 : Delay  DelayLength=6
  Out1 : Outport
  wires:
  In1/1 -> multiplier/1
  In2/1 -> multiplier/2
  multiplier/1 -> multiplier_pd1/1
  multiplier_pd1/1 -> Out1/1

== system gm_parallel_phase_voltages_per_switching_state_6/Phase_voltages_per_switching_state/Subsystem/MATLAB Function13/multiplier1 ==
  In1 : Inport
  In2 : Inport  Port=2
  multiplier1 : Product  Inputs=**  OutDataTypeStr=single  SampleTime=1e-08
  multiplier1_pd1 : Delay  DelayLength=6
  Out1 : Outport
  wires:
  In1/1 -> multiplier1/1
  In2/1 -> multiplier1/2
  multiplier1/1 -> multiplier1_pd1/1
  multiplier1_pd1/1 -> Out1/1

== system gm_parallel_phase_voltages_per_switching_state_6/Phase_voltages_per_switching_state/Subsystem/MATLAB Function13/multiplier2 ==
  In1 : Inport
  In2 : Inport  Port=2
  multiplier2 : Product  Inputs=**  OutDataTypeStr=single  SampleTime=1e-08
  multiplier2_pd1 : Delay  DelayLength=6
  Out1 : Outport
  wires:
  In1/1 -> multiplier2/1
  In2/1 -> multiplier2/2
  multiplier2/1 -> multiplier2_pd1/1
  multiplier2_pd1/1 -> Out1/1

== system gm_parallel_phase_voltages_per_switching_state_6/Phase_voltages_per_switching_state/Subsystem/MATLAB Function13/multiplier3 ==
  In1 : Inport
  In2 : Inport  Port=2
  multiplier3 : Product  Inputs=**  OutDataTypeStr=single  SampleTime=1e-08
  multiplier3_pd1 : Delay  DelayLength=6
  Out1 : Outport
  wires:
  In1/1 -> multiplier3/1
  In2/1 -> multiplier3/2
  multiplier3/1 -> multiplier3_pd1/1
  multiplier3_pd1/1 -> Out1/1

== system gm_parallel_phase_voltages_per_switching_state_6/Phase_voltages_per_switching_state/Subsystem/MATLAB Function13/multiplier4 ==
  In1 : Inport
  In2 : Inport  Port=2
  multiplier4 : Product  Inputs=**  OutDataTypeStr=single  SampleTime=1e-08
  multiplier4_pd1 : Delay  DelayLength=6
  Out1 : Outport
  wires:
  In1/1 -> multiplier4/1
  In2/1 -> multiplier4/2
  multiplier4/1 -> multiplier4_pd1/1
  multiplier4_pd1/1 -> Out1/1

== system gm_parallel_phase_voltages_per_switching_state_6/Phase_voltages_per_switching_state/Subsystem/MATLAB Function13/uminus ==
  In1 : Inport
  uminus : UnaryMinus  SampleTime=1e-08
  Out1 : Outport
  wires:
  In1/1 -> uminus/1
  uminus/1 -> Out1/1

== system gm_parallel_phase_voltages_per_switching_state_6/Phase_voltages_per_switching_state/Subsystem/MATLAB Function14/adder1 ==
  In1 : Inport
  In2 : Inport  Port=2
  adder1 : Sum  OutDataTypeStr=single  SampleTime=1e-08
  adder1_pd1 : Delay  DelayLength=6
  Out1 : Outport
  wires:
  In1/1 -> adder1/1
  In2/1 -> adder1/2
  adder1/1 -> adder1_pd1/1
  adder1_pd1/1 -> Out1/1

== system gm_parallel_phase_voltages_per_switching_state_6/Phase_voltages_per_switching_state/Subsystem/MATLAB Function14/adder2 ==
  In1 : Inport
  In2 : Inport  Port=2
  adder2 : Sum  OutDataTypeStr=single  SampleTime=1e-08
  adder2_pd1 : Delay  DelayLength=6
  Out1 : Outport
  wires:
  In1/1 -> adder2/1
  In2/1 -> adder2/2
  adder2/1 -> adder2_pd1/1
  adder2_pd1/1 -> Out1/1

== system gm_parallel_phase_voltages_per_switching_state_6/Phase_voltages_per_switching_state/Subsystem/MATLAB Function14/cos_to_sincos ==
  In1 : Inport
  cos_to_sincos : Trigonometry  Operator=sincos  SampleTime=1e-08
  cos_to_sincos_pd1 : Delay  DelayLength=27
  cos_to_sincos_pd2 : Delay  DelayLength=27
  Out1 : Outport
  Out2 : Outport  Port=2
  wires:
  In1/1 -> cos_to_sincos/1
  cos_to_sincos/1 -> cos_to_sincos_pd1/1
  cos_to_sincos_pd1/1 -> Out1/1
  cos_to_sincos/2 -> cos_to_sincos_pd2/1
  cos_to_sincos_pd2/1 -> Out2/1

== system gm_parallel_phase_voltages_per_switching_state_6/Phase_voltages_per_switching_state/Subsystem/MATLAB Function14/multiplier ==
  In1 : Inport
  In2 : Inport  Port=2
  multiplier : Product  Inputs=**  OutDataTypeStr=single  SampleTime=1e-08
  multiplier_pd1 : Delay  DelayLength=6
  Out1 : Outport
  wires:
  In1/1 -> multiplier/1
  In2/1 -> multiplier/2
  multiplier/1 -> multiplier_pd1/1
  multiplier_pd1/1 -> Out1/1

== system gm_parallel_phase_voltages_per_switching_state_6/Phase_voltages_per_switching_state/Subsystem/MATLAB Function14/multiplier1 ==
  In1 : Inport
  In2 : Inport  Port=2
  multiplier1 : Product  Inputs=**  OutDataTypeStr=single  SampleTime=1e-08
  multiplier1_pd1 : Delay  DelayLength=6
  Out1 : Outport
  wires:
  In1/1 -> multiplier1/1
  In2/1 -> multiplier1/2
  multiplier1/1 -> multiplier1_pd1/1
  multiplier1_pd1/1 -> Out1/1

== system gm_parallel_phase_voltages_per_switching_state_6/Phase_voltages_per_switching_state/Subsystem/MATLAB Function14/multiplier2 ==
  In1 : Inport
  In2 : Inport  Port=2
  multiplier2 : Product  Inputs=**  OutDataTypeStr=single  SampleTime=1e-08
  multiplier2_pd1 : Delay  DelayLength=6
  Out1 : Outport
  wires:
  In1/1 -> multiplier2/1
  In2/1 -> multiplier2/2
  multiplier2/1 -> multiplier2_pd1/1
  multiplier2_pd1/1 -> Out1/1

== system gm_parallel_phase_voltages_per_switching_state_6/Phase_voltages_per_switching_state/Subsystem/MATLAB Function14/multiplier3 ==
  In1 : Inport
  In2 : Inport  Port=2
  multiplier3 : Product  Inputs=**  OutDataTypeStr=single  SampleTime=1e-08
  multiplier3_pd1 : Delay  DelayLength=6
  Out1 : Outport
  wires:
  In1/1 -> multiplier3/1
  In2/1 -> multiplier3/2
  multiplier3/1 -> multiplier3_pd1/1
  multiplier3_pd1/1 -> Out1/1

== system gm_parallel_phase_voltages_per_switching_state_6/Phase_voltages_per_switching_state/Subsystem/MATLAB Function14/multiplier4 ==
  In1 : Inport
  In2 : Inport  Port=2
  multiplier4 : Product  Inputs=**  OutDataTypeStr=single  SampleTime=1e-08
  multiplier4_pd1 : Delay  DelayLength=6
  Out1 : Outport
  wires:
  In1/1 -> multiplier4/1
  In2/1 -> multiplier4/2
  multiplier4/1 -> multiplier4_pd1/1
  multiplier4_pd1/1 -> Out1/1

== system gm_parallel_phase_voltages_per_switching_state_6/Phase_voltages_per_switching_state/Subsystem/MATLAB Function14/uminus ==
  In1 : Inport
  uminus : UnaryMinus  SampleTime=1e-08
  Out1 : Outport
  wires:
  In1/1 -> uminus/1
  uminus/1 -> Out1/1

== system gm_parallel_phase_voltages_per_switching_state_6/Phase_voltages_per_switching_state/Subsystem/MATLAB Function15/adder1 ==
  In1 : Inport
  In2 : Inport  Port=2
  adder1 : Sum  OutDataTypeStr=single  SampleTime=1e-08
  adder1_pd1 : Delay  DelayLength=6
  Out1 : Outport
  wires:
  In1/1 -> adder1/1
  In2/1 -> adder1/2
  adder1/1 -> adder1_pd1/1
  adder1_pd1/1 -> Out1/1
